simulink model "untitled"  (R2022b)
settings: Solver=VariableStepAuto  StartTime=0.0  StopTime=10.0  RelTol=1e-3
settings Model: Creator=LiNing  LastModifiedBy=LiNing

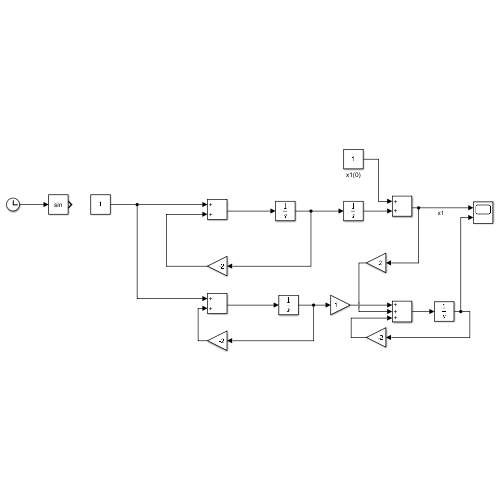
[thumbnail: Simulink's stored preview of the top-level diagram]
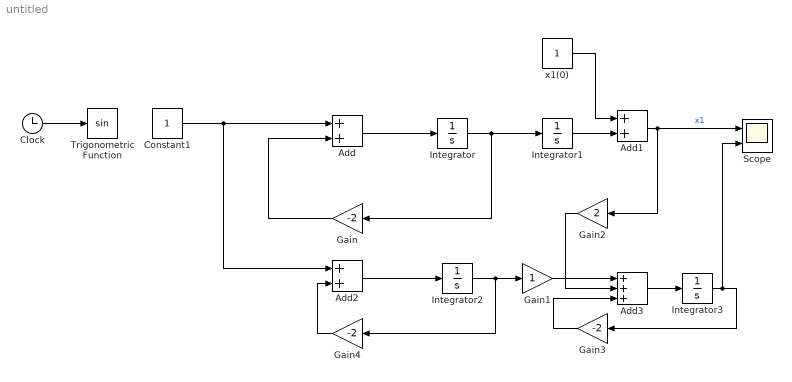
== system untitled ==
  Add : Sum
  Add1 : Sum
  Add2 : Sum
  Add3 : Sum  Inputs=+++
  Clock : Clock
  Constant1 : Constant
  Gain : Gain  Gain=-2
  Gain1 : Gain
  Gain2 : Gain  Gain=2
  Gain3 : Gain  Gain=-2
  Gain4 : Gain  Gain=-2
  Integrator{,1..3} (4 alike) : Integrator
  Scope : Scope  NumInputPorts=2
  Trigonometric Function : Trigonometry
  x1(0) : Constant
  wires:
  Gain/1 -> Add/2
  Add/1 -> Integrator/1
  Integrator/1 -> Gain/1, Integrator1/1
  Integrator1/1 -> Add1/2
  x1(0)/1 -> Add1/1
  Add1/1 -> Gain2/1, Scope/1  "x1"
  Clock/1 -> Trigonometric Function/1
  Gain4/1 -> Add2/2
  Add2/1 -> Integrator2/1
  Integrator2/1 -> Gain4/1, Gain1/1
  Gain1/1 -> Add3/1
  Gain2/1 -> Add3/2
  Gain3/1 -> Add3/3
  Add3/1 -> Integrator3/1
  Integrator3/1 -> Scope/2, Gain3/1
  Constant1/1 -> Add2/1, Add/1
